simulink model "AXON_Kinematics_CONF5"  (R2019b)
settings: Solver=ode4  StartTime=0.0  StopTime=80  FixedStep=0.025  RelTol=1e-3  EnableMultiTasking=on
InitFcn:
  | Ref_Path3;
  | roboparam;
StopFcn:
  | figure(1)
  | plot(xy_axon.DATA(:,1),xy_axon.DATA(:,2),'red')
  | hold on
  | plot(xy_trolley.DATA(:,1),xy_trolley.DATA(:,2),'green')
  | legend('Reference trajectory', 'Robot trajectory', 'Trailer trajectory')
values from neighbouring files (symbols this model uses):
  th0 = z(4)    [AXON_Dynamics_CONF5_vw_old.m]    (also in AllInOneDynamic.m = th(i,2); Kinematics.m; PathGenerationPlotting_Dynamics.m = th(i,2); PathGenerationPlotting_Kinematics.m = z(i,4))
  xaxon0 = xtrolley0+rho1*cos(th1)+rho0*cos(th0)    [roboparam.m]
  yaxon0 = ytrolley0+rho1*sin(th1)+rho0*sin(th0)    [roboparam.m]
settings Model: Creator=e0010448  LastModifiedBy=vladkhon
settings DataIOCC: LimitDataPoints=on  SaveFormat=StructureWithTime  ReturnWorkspaceOutputs=off
settings OptimizationCC: BlockReduction=off  BufferReuse=off  LifeSpan=inf
settings DebuggingCC: AlgebraicLoopMsg=none  UnconnectedInputMsg=none  UnconnectedOutputMsg=none  UnconnectedLineMsg=none  AllowSymbolicDim=off  SFUnexpectedBacktrackingDiag=warning  SFNoUnconditionalDefaultTransitionDiag=warning  SFExecutionAtInitializationDiag=none  ArithmeticOperatorsInVariantConditions=warning
settings HardwareCC: ProdBitPerPointer=32  ProdBitPerSizeT=32  ProdBitPerPtrDiffT=32  ProdLargestAtomicFloat=None  ProdIntDivRoundTo=Undefined  ProdEndianess=Unspecified  ProdWordSize=32  ProdHWDeviceType=32-bit Generic
settings ModelReferenceCC: PropagateSignalLabelsOutOfModel=off
settings SFSimCC: SimUseLocalCustomCode=off  CustomCodeUndefinedFunction=UseInterfaceOnly
settings RTWCC: RTWUseLocalCustomCode=off
settings CodeAppCC: StateflowObjectComments=on
settings GRTTargetCC: TargetLangStandard=C89/C90 (ANSI)  GeneratePreprocessorConditionals=Disable all
settings ConfigComp: CovMetricSettings=dw  CovHtmlReporting=on  CovSaveCumulativeToWorkspaceVar=on  CovSaveSingleToWorkspaceVar=on  CovExternalEMLEnable=off

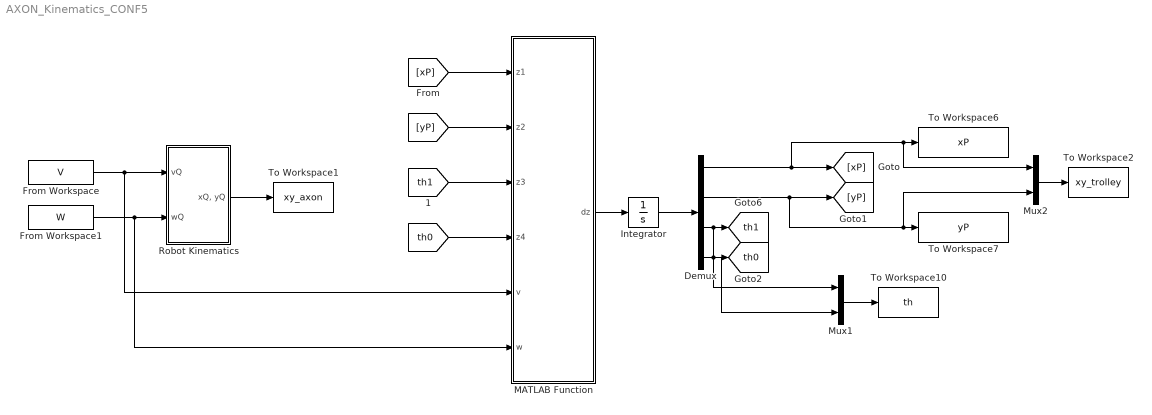
== system AXON_Kinematics_CONF5 ==
  Demux : Demux
  From Workspace : FromWorkspace  VariableName=V  SampleTime=0
  From Workspace1 : FromWorkspace  VariableName=W  SampleTime=0
  Integrator : Integrator  InitialCondition=[0 0 0 0]
  MATLAB Function : MATLAB Function  TreatAsAtomicUnit=on
  Mux1 : Mux  Inputs=2
  Mux2 : Mux  Inputs=2
  Robot Kinematics : Subsystem
  To Workspace1 : ToWorkspace  VariableName=xy_axon  SaveFormat=Timeseries  SampleTime=-1
  To Workspace10 : ToWorkspace  VariableName=th  SampleTime=-1
  To Workspace2 : ToWorkspace  VariableName=xy_trolley  SaveFormat=Timeseries  SampleTime=-1
  To Workspace6 : ToWorkspace  VariableName=xP  SampleTime=-1
  To Workspace7 : ToWorkspace  VariableName=yP  SampleTime=-1
  tag scope: th0=global, th1=global
  wires:
  Robot Kinematics/1("xQ, yQ") -> To Workspace1/1
  Mux1/1 -> To Workspace10/1
  From Workspace1/1 -> MATLAB Function/6(w), Robot Kinematics/2(wQ)
  [th0] -> MATLAB Function/4(z4)
  From Workspace/1 -> MATLAB Function/5(v), Robot Kinematics/1(vQ)
  Demux/1 -> Mux2/1, To Workspace6/1, [xP]
  Demux/2 -> Mux2/2, To Workspace7/1, [yP]
  [yP] -> MATLAB Function/2(z2)
  Demux/3 -> Mux1/1, [th1]
  MATLAB Function/1(dz) -> Integrator/1
  Demux/4 -> Mux1/2, [th0]
  [xP] -> MATLAB Function/1(z1)
  [th1] -> MATLAB Function/3(z3)
  Integrator/1 -> Demux/1
  Mux2/1 -> To Workspace2/1

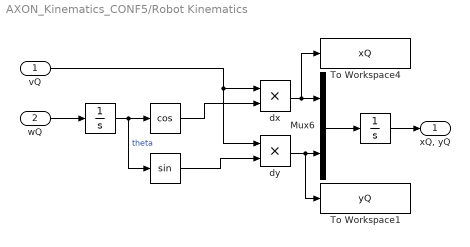
== system AXON_Kinematics_CONF5/Robot Kinematics ==
  vQ : Inport
  wQ : Inport  Port=2
  " " : Trigonometry  Operator=cos
  "  " : Trigonometry
  "   " : Integrator  InitialCondition=th0
  "    " : Integrator  InitialCondition=[xaxon0 yaxon0]
  Mux6 : Mux  Inputs=2
  To Workspace1 : ToWorkspace  VariableName=yQ  SampleTime=-1
  To Workspace4 : ToWorkspace  VariableName=xQ  SampleTime=-1
  dx : Product
  dy : Product
  "xQ, yQ" : Outport  VectorParamsAs1DForOutWhenUnconnected=off
  wires:
  dx/1 -> To Workspace4/1, Mux6/1
  dy/1 -> To Workspace1/1, Mux6/2
  vQ/1 -> dy/1, dx/1
  wQ/1 -> "   "/1
  " "/1 -> dx/2
  "   "/1 -> "  "/1, " "/1  "theta"
  "  "/1 -> dy/2
  Mux6/1 -> "    "/1
  "    "/1 -> "xQ, yQ"/1

== matlab function AXON_Kinematics_CONF5/MATLAB Function ==
  data: z1 input; dz output; z2 input; z3 input; z4 input; v input; w input
function dz = AXON_Dynamics_CONF5_VW_Simulink(z1,z2,z3,z4,v,w)
%% ODE function for the dynamics of configuration 5 that uses linear and angular velocity states
% t -> time variable
% z -> state variables  [x,y,th1,th0,psicw(4),v,w]

% variable state assignment

% position of pt P (x,y) axon orientation (th0) and trolley orientation (th1)
x = z1;
y = z2;
th1 = z3;
th0 = z4;

rho0 = 0.5;     % 0.5; 
rho1 = 1;       % distance in m

%% Config 5
%% Axon Kinematics
% dx, dy, dth1, dth0 -> change in position and orientation
dx = cos(th1)*cos(th1-th0)*v-cos(th1)*sin(th1-th0)*rho0*w;
dy = sin(th1)*cos(th1-th0)*v-sin(th1)*sin(th1-th0)*rho0*w;
dth1 = -sin(th1-th0)/rho1*v-(cos(th1-th0)*rho0)/rho1*w;
dth0 = w;

dz = [dx,dy,dth1,dth0].';
